simulink model "InvertedPD1"  (Simulink 5.0)
settings: Solver=ode1  SolverMode=SingleTasking  StartTime=0.0  StopTime=70.0  FixedStep=0.001  RelTol=1e-3
libraries: pci1711 x3
settings Model: LastModifiedBy=cedrics  ExtModeMexFile=rtwinext  ExtModeTrigMode=oneshot  ExtModeTrigDuration=100000  ExtModeLogAll=off  SimulationMode=external  LimitDataPoints=off  BlockReductionOpt=off  BooleanDataType=off  RTWSystemTargetFile=rtwinfbk.tlc  RTWTemplateMakefile=winfbktmf  RTWOptions="-aCCOptimize=1 -aEnforceIntegerDowncast=1 -aExtMode=1 -aFoldNonRolledExpr=1 -aForceParamTrailComments=0 -aGenerateComments=1 -aGenerateReport=0 -aIncDataTypeInIds=0 -aIncHierarchyInIds=0 -aInlineInvariantSignals=0 -aInlineParameters=0 -aInlinedPrmAccess=\"Literals\" -aLocalBlockOutputs=1 -aMaxRTWIdLen=31 -aPrefixModelToSubsysFcnNames=1 -aRTWVerbose=1 -aRebuildAll=0 -aRollThreshold=5 -aShowEliminatedStatements=1"

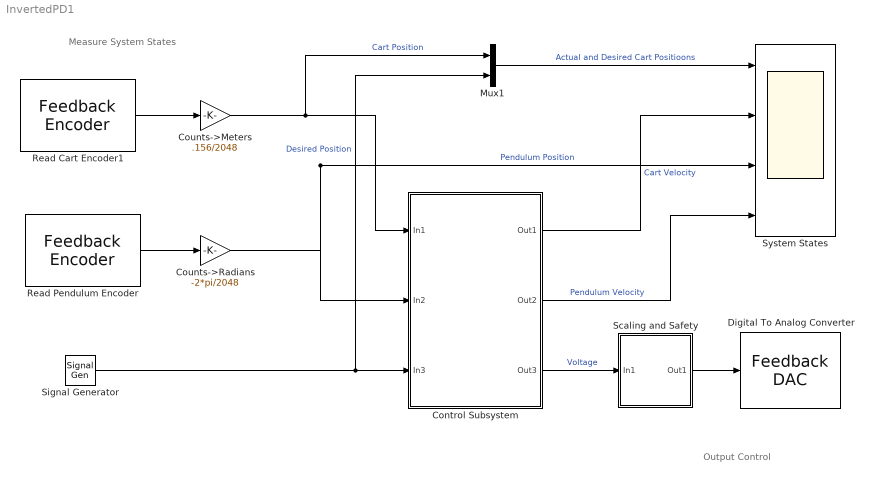
== system InvertedPD1 ==
  note: Measure System States
  note: Output Control
  Control Subsystem : Subsystem
  Counts->Meters : Gain  Gain=.156/2048  SaturateOnIntegerOverflow=on
  Counts->Radians : Gain  Gain=-2*pi/2048  SaturateOnIntegerOverflow=on
  Digital To Analog Converter : pci1711/Advantech  PCI1711 I//O Board Lib/Feedback DAC  channel=0  range=0  tsamp=0.001  hwAccess=on
  Mux1 : Mux  Inputs=2
  Read Cart Encoder1 : pci1711/Advantech  PCI1711 I//O Board Lib/Feedback Encoder   channel=0  offset=0  tsamp=0.001  hwAccess=on
  Read Pendulum Encoder : pci1711/Advantech  PCI1711 I//O Board Lib/Feedback Encoder   channel=1  offset=-1024  tsamp=0.001  hwAccess=on
  Scaling and Safety : Subsystem
  Signal Generator : SignalGenerator  Amplitude=0.1  Frequency=0.1
  System States : Scope  NumInputPorts=4
      settings: TimeRange=70  YMin=-0.5~-1~-6~-15  YMax=0.5~1~6~15  Decimation=0.1  SampleInput=on  SampleTime=0.01
  wires:
  Counts->Meters/1 -> Mux1/1, Control Subsystem/1(In1)  "Cart Position"
  Counts->Radians/1 -> System States/3, Control Subsystem/2(In2)  "Pendulum Position"
  Scaling and Safety/1(Out1) -> Digital To Analog Converter/1
  Signal Generator/1 -> Mux1/2, Control Subsystem/3(In3)  "Desired Position"
  Control Subsystem/3(Out3) -> Scaling and Safety/1(In1)  "Voltage"
  Mux1/1 -> System States/1  "Actual and Desired Cart Positioons"
  Read Cart Encoder1/1 -> Counts->Meters/1
  Read Pendulum Encoder/1 -> Counts->Radians/1
  Control Subsystem/1(Out1) -> System States/2  "Cart Velocity"
  Control Subsystem/2(Out2) -> System States/4  "Pendulum Velocity"

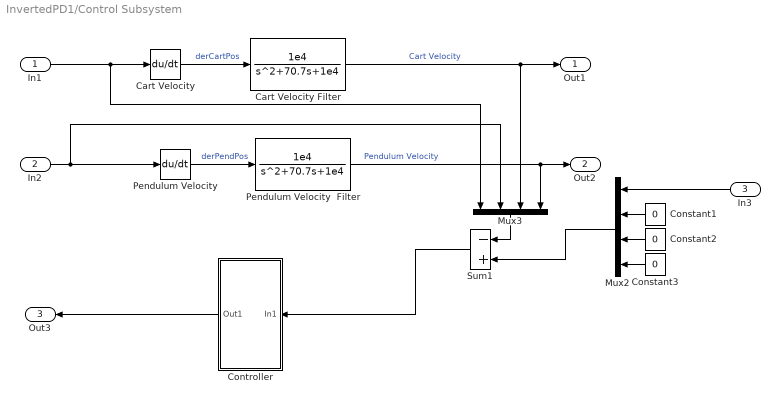
== system InvertedPD1/Control Subsystem ==
  In1 : Inport
  In2 : Inport  Port=2
  In3 : Inport  Orientation=left  Port=3
  Cart Velocity : Derivative
  Cart Velocity Filter : TransferFcn  Numerator=[1e4]  Denominator=[1 70.7 1e4]
  Constant1 : Constant  Orientation=left  Value=0
  Constant2 : Constant  Orientation=left  Value=0
  Constant3 : Constant  Orientation=left  Value=0
  Controller : Subsystem  Orientation=left
  Mux2 : Mux  Orientation=left
  Mux3 : Mux  Orientation=down
  Pendulum Velocity : Derivative
  Pendulum Velocity  Filter : TransferFcn  Numerator=[1e4]  Denominator=[1 70.7 1e4]
  Sum1 : Sum  Orientation=left  Inputs=-+  SaturateOnIntegerOverflow=on  InputSameDT=on
  Out1 : Outport
  Out2 : Outport  Port=2
  Out3 : Outport  Orientation=left  Port=3
  wires:
  Cart Velocity/1 -> Cart Velocity Filter/1  "derCartPos"
  Pendulum Velocity/1 -> Pendulum Velocity  Filter/1  "derPendPos"
  Cart Velocity Filter/1 -> Mux3/3, Out1/1  "Cart Velocity"
  Pendulum Velocity  Filter/1 -> Mux3/4, Out2/1  "Pendulum Velocity"
  Mux2/1 -> Sum1/2
  Constant1/1 -> Mux2/2
  Constant2/1 -> Mux2/3
  Constant3/1 -> Mux2/4
  Mux3/1 -> Sum1/1
  In1/1 -> Cart Velocity/1, Mux3/1
  In2/1 -> Pendulum Velocity/1, Mux3/2
  In3/1 -> Mux2/1
  Controller/1(Out1) -> Out3/1
  Sum1/1 -> Controller/1(In1)

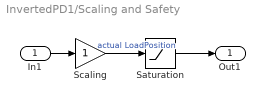
== system InvertedPD1/Scaling and Safety ==
  In1 : Inport
  Saturation : Saturate  UpperLimit=2.5  LowerLimit=-2.5
  Scaling : Gain  SaturateOnIntegerOverflow=on
  Out1 : Outport
  wires:
  Saturation/1 -> Out1/1
  In1/1 -> Scaling/1
  Scaling/1 -> Saturation/1  "actual LoadPosition"

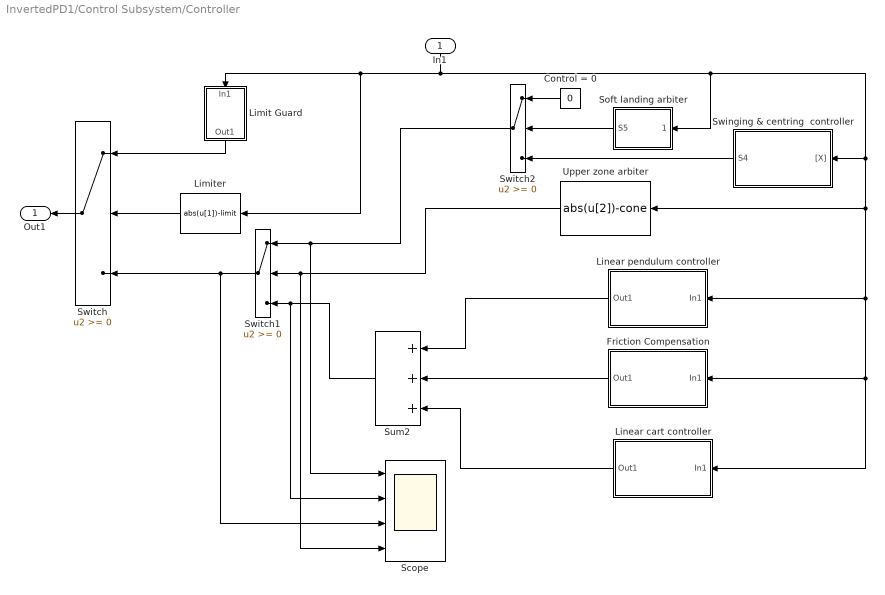
== system InvertedPD1/Control Subsystem/Controller ==
  In1 : Inport  Orientation=down
  Control = 0 : Constant  Orientation=left  Value=0
  Friction Compensation : Subsystem  Orientation=left  mask(linear){frictionCompNeg=.1, frictionCompPos=.1}
      mask prompts: frictionCompNeg "Friction Compensation Magnitude in Negative Direction"; frictionCompPos "Friction Compensation Magnitude in Positive Direction"
      mask Display: plot(0,0,100,100,[40,30,20],[87,85,80],[46,54,54,46,46],[90,90,80,80,90],[46,45,45,46,54,55,55,54,46],[78,80,90,91,91,90,80,78,78],[51,51,49,49],[78,10,10,78],[90,80,70,60],[70,80,85,88],[20,10],[80,70],[20,20,15],[73,80,80],[85,80,80],[80,80,74])
  Limit Guard : Subsystem  Orientation=down  mask{umax2=.5}
      mask prompts: umax2 "maximal force"
      mask Display: plot(0,0,100,100,[20,40,40,20,20],[60,60,49,49,60],[56,59,40],[58,55,55],[56,59],[52,55],[38,13,13],[39,39,46],[46,13],[46,46],[23,23,24,22,24,24,22,23],[47,45,49,48,48,46,47,49],[36,35,34,34,37,34,36,35,36,37,35,34,35],[49,48,46,49,48,47,45,47,48,46,46,47,49],[22,22,24,24],[46,49,48,47])
  Limiter : Fcn  Orientation=left  Expr=abs(u[1])-limit  mask{limit=0.3}
      mask prompts: limit "Rail mg - rail limit"
      mask Display: plot(0,0,100,100,[10,90,90,10],[52,52,50,50],[30,30],[52,60],[70,68,68,70,70],[60,60,52,52,60],[30,32,32,30],[52,52,60,60])
  Linear cart controller : Subsystem  Orientation=left  mask(linear){K1=-7, K3=-4}
      mask prompts: K1 "K1  - position  feedback"; K3 "K3  -  velocity  feedback"
      mask Display: plot(0,0,100,100,[40,30,20],[87,85,80],[46,54,54,46,46],[90,90,80,80,90],[46,45,45,46,54,55,55,54,46],[78,80,90,91,91,90,80,78,78],[51,51,49,49],[78,10,10,78],[90,80,70,60],[70,80,85,88],[20,10],[80,70],[20,20,15],[73,80,80],[85,80,80],[80,80,74])
  Linear pendulum controller : Subsystem  Orientation=left  mask(linear){K2=50, K4=3.5}
      mask prompts: K2 "K2  - angle  feedback"; K4 "K4  - angular velocity  feedback"
      mask Display: plot(0,0,100,100,[40,30,20],[87,85,80],[46,54,54,46,46],[90,90,80,80,90],[46,45,45,46,54,55,55,54,46],[78,80,90,91,91,90,80,78,78],[51,51,49,49],[78,10,10,78],[90,80,70,60],[70,80,85,88],[20,10],[80,70],[20,20,15],[73,80,80],[85,80,80],[80,80,74])
  Scope : Scope  NumInputPorts=4
      settings: YMin=-5~-5~-5~-5  YMax=5~5~5~5
  Soft landing arbiter : Subsystem  Orientation=left  mask(Soft landing){k=8.6, R=0.35}
      mask prompts: k "k coefficient"; R "R value"
      mask help: Soft landing
      mask Display: plot(0,0,100,100,[14,20,20,14,14],[20,20,8,8,20],[40,35,35,40,40],[39,40,51,51,40],[60,55,55,56,60,60],[70,70,60,60,60,71],[74,74,80,80,74],[80,91,91,80,80])
  Sum2 : Sum  Orientation=left  Inputs=+++  SaturateOnIntegerOverflow=on  InputSameDT=on
  Swinging & centring  controller : Subsystem  Orientation=left  mask(swing){umax=1, alfa=2.2, beta=.4, gamma=0.}
      mask prompts: umax "maximal control umax"; alfa "ALPHA - centering cart factor related to position"; beta "BETA - centering cart factor related to velocity"; gamma "GAMMA - centering cart factor related to + - pi/2 angle"
      mask help: swing
      mask Display: plot(0,0,100,100,[20,20],[12,87],[93,90,90,93,7],[50,46,54,50,50],[20,22,18,20],[87,80,80,88],[80,80,75,75,71,71,65,65,60,60,49,49,40,40,20],[50,40,40,60,60,50,50,80,80,20,21,80,80,21,20])
  Switch : Switch  Orientation=left  SaturateOnIntegerOverflow=on  InputSameDT=on
  Switch1 : Switch  Orientation=left  SaturateOnIntegerOverflow=on  InputSameDT=on
  Switch2 : Switch  Orientation=left  SaturateOnIntegerOverflow=on  InputSameDT=on
  Upper zone arbiter : Fcn  Orientation=left  Expr=abs(u[2])-cone  mask(ZONE){cone=0.3}
      mask prompts: cone "Stab.zone - width of stabilization zone [rad]"
      mask help: ZONE
      mask Display: plot(0,0,100,100,[40,60,80,83,80,60,40,20,17,20,40],[89,89,80,70,60,51,51,60,69,80,90],[83,50,17],[70,8,68])
  Out1 : Outport  Orientation=left
  wires:
  Swinging & centring  controller/1(S4) -> Switch2/3
  Soft landing arbiter/1(S5) -> Switch2/2
  Limiter/1 -> Switch/2
  Control = 0/1 -> Switch2/1
  Linear pendulum controller/1(Out1) -> Sum2/1
  Linear cart controller/1(Out1) -> Sum2/3
  Friction Compensation/1(Out1) -> Sum2/2
  Switch2/1 -> Switch1/1, Scope/1
  Sum2/1 -> Switch1/3, Scope/2
  Upper zone arbiter/1 -> Switch1/2, Scope/4
  Limit Guard/1(Out1) -> Switch/1
  Switch1/1 -> Scope/3, Switch/3
  In1/1 -> Soft landing arbiter/1((x1,x2,x3,x4)), Upper zone arbiter/1, Linear pendulum controller/1(In1), Linear cart controller/1(In1), Friction Compensation/1(In1), Swinging & centring  controller/1("[X]"), Limiter/1, Limit Guard/1(In1)
  Switch/1 -> Out1/1

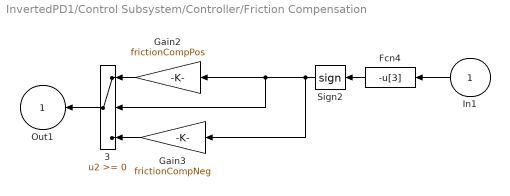
== system InvertedPD1/Control Subsystem/Controller/Friction Compensation ==
  In1 : Inport  Orientation=left
  3 : Switch  Orientation=left  SaturateOnIntegerOverflow=on  InputSameDT=on
  Fcn4 : Fcn  Orientation=left  Expr=-u[3]
  Gain2 : Gain  Orientation=left  Gain=frictionCompPos  SaturateOnIntegerOverflow=on
  Gain3 : Gain  Orientation=left  Gain=frictionCompNeg  SaturateOnIntegerOverflow=on
  Sign2 : Signum  Tag=T  Orientation=left
  Out1 : Outport  Orientation=left  InitialOutput=0
  wires:
  Fcn4/1 -> Sign2/1
  In1/1 -> Fcn4/1
  Gain2/1 -> 3/1
  Gain3/1 -> 3/3
  Sign2/1 -> Gain3/1, Gain2/1, 3/2
  3/1 -> Out1/1

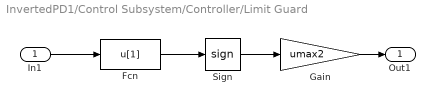
== system InvertedPD1/Control Subsystem/Controller/Limit Guard ==
  In1 : Inport
  Fcn : Fcn  Expr=u[1]
  Gain : Gain  Gain=umax2  SaturateOnIntegerOverflow=on
  Sign : Signum
  Out1 : Outport  InitialOutput=0
  wires:
  Sign/1 -> Gain/1
  Gain/1 -> Out1/1
  Fcn/1 -> Sign/1
  In1/1 -> Fcn/1

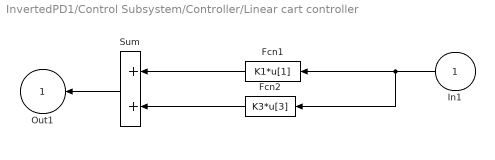
== system InvertedPD1/Control Subsystem/Controller/Linear cart controller ==
  In1 : Inport  Orientation=left
  Fcn1 : Fcn  Orientation=left  Expr=K1*u[1]
  Fcn2 : Fcn  Orientation=left  Expr=K3*u[3]
  Sum : Sum  Orientation=left  SaturateOnIntegerOverflow=on  InputSameDT=on
  Out1 : Outport  Orientation=left  InitialOutput=0
  wires:
  Fcn1/1 -> Sum/1
  Fcn2/1 -> Sum/2
  Sum/1 -> Out1/1
  In1/1 -> Fcn1/1, Fcn2/1

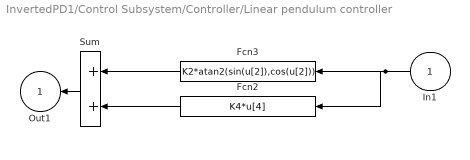
== system InvertedPD1/Control Subsystem/Controller/Linear pendulum controller ==
  In1 : Inport  Orientation=left
  Fcn2 : Fcn  Orientation=left  Expr=K4*u[4]
  Fcn3 : Fcn  Orientation=left  Expr=K2*atan2(sin(u[2]),cos(u[2]))
  Sum : Sum  Orientation=left  SaturateOnIntegerOverflow=on  InputSameDT=on
  Out1 : Outport  Orientation=left  InitialOutput=0
  wires:
  Sum/1 -> Out1/1
  Fcn2/1 -> Sum/2
  In1/1 -> Fcn2/1, Fcn3/1
  Fcn3/1 -> Sum/1

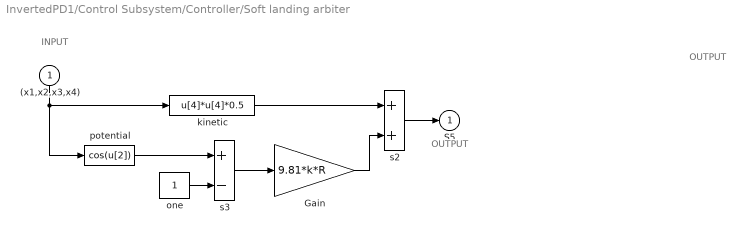
== system InvertedPD1/Control Subsystem/Controller/Soft landing arbiter ==
  note: OUTPUT
  note: OUTPUT
  note: INPUT
  (x1,x2,x3,x4) : Inport  Orientation=down
  Gain : Gain  Gain=9.81*k*R  SaturateOnIntegerOverflow=on
  kinetic : Fcn  Expr=u[4]*u[4]*0.5
  "one " : Constant
  potential : Fcn  Expr=cos(u[2])
  s2 : Sum  SaturateOnIntegerOverflow=on  InputSameDT=on
  s3 : Sum  Inputs=+-  SaturateOnIntegerOverflow=on  InputSameDT=on
  S5 : Outport  InitialOutput=0
  wires:
  potential/1 -> s3/1
  "one "/1 -> s3/2
  kinetic/1 -> s2/1
  s3/1 -> Gain/1
  Gain/1 -> s2/2
  (x1,x2,x3,x4)/1 -> potential/1, kinetic/1
  s2/1 -> S5/1

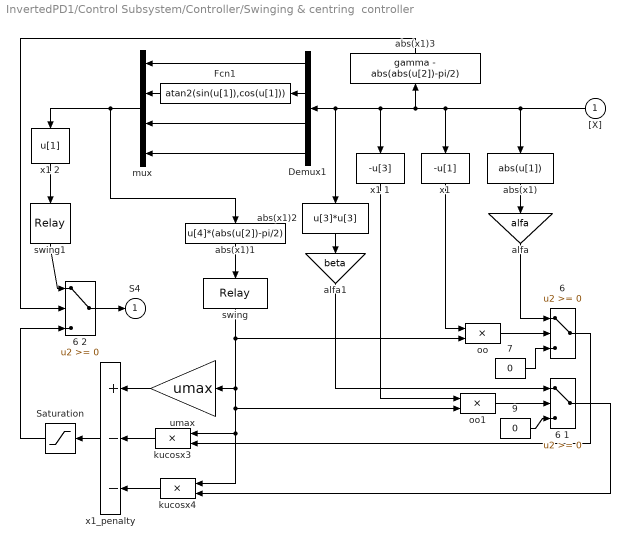
== system InvertedPD1/Control Subsystem/Controller/Swinging & centring  controller ==
  "[X]" : Inport  Orientation=left
  "6 " : Switch  SaturateOnIntegerOverflow=on  InputSameDT=on
  6 1 : Switch  SaturateOnIntegerOverflow=on  InputSameDT=on
  6 2 : Switch  SaturateOnIntegerOverflow=on  InputSameDT=on
  7 : Constant  Value=0
  9 : Constant  Value=0
  Demux1 : Demux  Orientation=left
  Fcn1 : Fcn  Orientation=left  Expr=atan2(sin(u[1]),cos(u[1]))
  Saturation : Saturate  Orientation=left  UpperLimit=umax  LowerLimit=-umax
  abs(x1) : Fcn  Orientation=down  Expr=abs(u[1])
  abs(x1)1 : Fcn  Orientation=down  Expr=u[4]*(abs(u[2])-pi/2)
  abs(x1)2 : Fcn  Orientation=down  Expr=u[3]*u[3]
  abs(x1)3 : Fcn  Orientation=up  Expr=gamma - abs(abs(u[2])-pi/2)
  alfa : Gain  Orientation=down  Gain=alfa  SaturateOnIntegerOverflow=on
  alfa1 : Gain  Orientation=down  Gain=beta  SaturateOnIntegerOverflow=on
  kucosx3 : Product  Orientation=left  SaturateOnIntegerOverflow=on  InputSameDT=on
  kucosx4 : Product  Orientation=left  SaturateOnIntegerOverflow=on  InputSameDT=on
  mux : Mux  Orientation=left
  oo : Product  SaturateOnIntegerOverflow=on  InputSameDT=on
  oo1 : Product  SaturateOnIntegerOverflow=on  InputSameDT=on
  swing : Relay  Orientation=down  OffOutputValue=-1
  swing1 : Relay  Orientation=down  OffOutputValue=-1
  umax : Gain  Orientation=left  Gain=umax  SaturateOnIntegerOverflow=on
  "x1 " : Fcn  Orientation=down  Expr=-u[1]
  x1 1 : Fcn  Orientation=down  Expr=-u[3]
  x1 2 : Fcn  Orientation=down  Expr=u[1]
  x1_penalty : Sum  Orientation=left  Inputs=+--  SaturateOnIntegerOverflow=on  InputSameDT=on
  S4 : Outport  InitialOutput=0
  wires:
  abs(x1)3/1 -> 6 2/2
  Demux1/4 -> mux/4
  Demux1/3 -> mux/3
  Demux1/1 -> mux/1
  Fcn1/1 -> mux/2
  Demux1/2 -> Fcn1/1
  x1_penalty/1 -> Saturation/1
  umax/1 -> x1_penalty/1
  kucosx3/1 -> x1_penalty/2
  oo/1 -> "6 "/2
  "6 "/1 -> kucosx3/2
  abs(x1)/1 -> alfa/1
  abs(x1)1/1 -> swing/1
  "[X]"/1 -> "x1 "/1, x1 1/1, Demux1/1, abs(x1)2/1, abs(x1)3/1, abs(x1)/1
  swing/1 -> umax/1, oo1/2, kucosx3/1, kucosx4/1, oo/2
  alfa/1 -> "6 "/1
  "x1 "/1 -> oo/1
  oo1/1 -> 6 1/2
  alfa1/1 -> 6 1/1
  x1 1/1 -> oo1/1
  abs(x1)2/1 -> alfa1/1
  kucosx4/1 -> x1_penalty/3
  6 1/1 -> kucosx4/2
  7/1 -> "6 "/3
  9/1 -> 6 1/3
  6 2/1 -> S4/1
  Saturation/1 -> 6 2/3
  x1 2/1 -> swing1/1
  mux/1 -> abs(x1)1/1, x1 2/1
  swing1/1 -> 6 2/1
